simulink model "UiRlab6_model3"  (R2021a)
settings: Solver=VariableStepAuto  StartTime=0.0  StopTime=40e-3  RelTol=1e-3
undefined symbols (not defined in the file): K, Ka, Kf, Ki, Komega, Kria, Krsim, Kt, Ktr, Kzi, Ta, Tf_sim, Ti, Tii, Tisim, Tomega, Tt, Ttr, Tzi
settings Model: Creator=Luka  LastModifiedBy=Luka

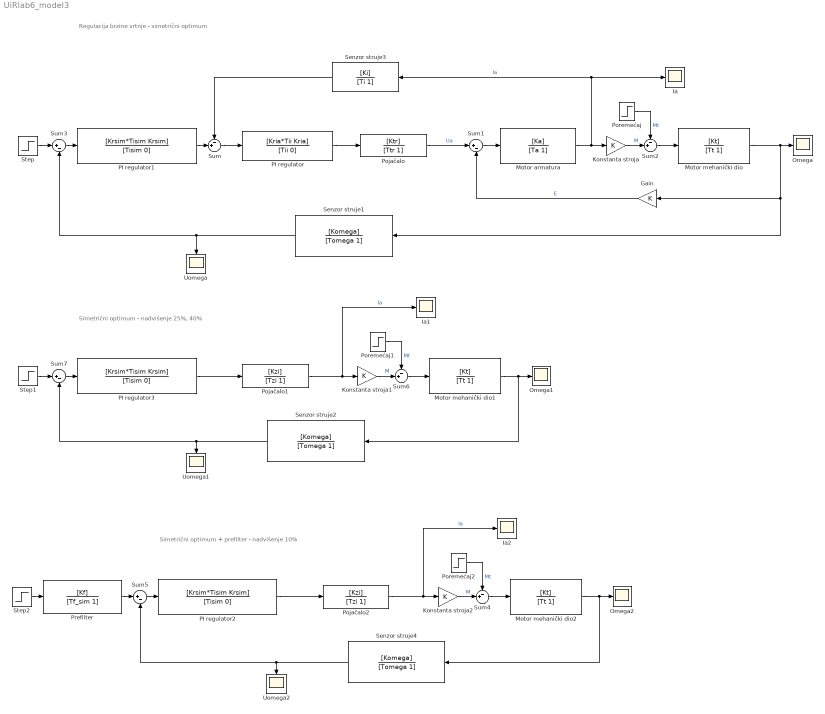
== system UiRlab6_model3 ==
  note: Simetrični optimum + prefilter - nadvišenje 10%
  note: Regulacija brzine vrtnje - simetrični optimum
  note: Simetrični optimum - nadvišenje 25%, 40%
  Gain : Gain  Gain=K
  Ia : Scope
  Ia1 : Scope
  Ia2 : Scope
  Konstanta stroja : Gain  Gain=K
  Konstanta stroja1 : Gain  Gain=K
  Konstanta stroja2 : Gain  Gain=K
  Motor armatura : TransferFcn  Numerator=[Ka]  Denominator=[Ta 1]
  Motor mehanički dio : TransferFcn  Numerator=[Kt]  Denominator=[Tt 1]
  Motor mehanički dio1 : TransferFcn  Numerator=[Kt]  Denominator=[Tt 1]
  Motor mehanički dio2 : TransferFcn  Numerator=[Kt]  Denominator=[Tt 1]
  Omega : Scope
  Omega1 : Scope
  Omega2 : Scope
  PI regulator : TransferFcn  Numerator=[Kria*Tii Kria]  Denominator=[Tii 0]
  PI regulator1 : TransferFcn  Numerator=[Krsim*Tisim Krsim]  Denominator=[Tisim 0]
  PI regulator2 : TransferFcn  Numerator=[Krsim*Tisim Krsim]  Denominator=[Tisim 0]
  PI regulator3 : TransferFcn  Numerator=[Krsim*Tisim Krsim]  Denominator=[Tisim 0]
  Pojačalo : TransferFcn  Numerator=[Ktr]  Denominator=[Ttr 1]
  Pojačalo1 : TransferFcn  Numerator=[Kzi]  Denominator=[Tzi 1]
  Pojačalo2 : TransferFcn  Numerator=[Kzi]  Denominator=[Tzi 1]
  Poremećaj : Step  Time=0  After=0  SampleTime=0
  Poremećaj1 : Step  Time=0  After=0  SampleTime=0
  Poremećaj2 : Step  Time=0  After=0  SampleTime=0
  Prefilter : TransferFcn  Numerator=[Kf]  Denominator=[Tf_sim 1]
  Senzor struje1 : TransferFcn  Numerator=[Komega]  Denominator=[Tomega 1]
  Senzor struje2 : TransferFcn  Numerator=[Komega]  Denominator=[Tomega 1]
  Senzor struje3 : TransferFcn  Numerator=[Ki]  Denominator=[Ti 1]
  Senzor struje4 : TransferFcn  Numerator=[Komega]  Denominator=[Tomega 1]
  Step : Step  Time=0  After=0.1  SampleTime=0
  Step1 : Step  Time=0  After=0.1  SampleTime=0
  Step2 : Step  Time=0  After=0.1  SampleTime=0
  Sum{,2,4,6} (4 alike) : Sum  Inputs=-+|
  Sum{1,3,5,7} (4 alike) : Sum  Inputs=|+-
  Uomega : Scope
  Uomega1 : Scope
  Uomega2 : Scope
  wires:
  Pojačalo1/1 -> Ia1/1, Konstanta stroja1/1  "Ia"
  Senzor struje1/1 -> Sum3/2, Uomega/1
  Step/1 -> Sum3/1
  PI regulator1/1 -> Sum/2
  Motor mehanički dio/1 -> Senzor struje1/1, Gain/1, Omega/1
  Konstanta stroja/1 -> Sum2/2  "M"
  Sum3/1 -> PI regulator1/1
  Senzor struje3/1 -> Sum/1
  PI regulator/1 -> Pojačalo/1
  Prefilter/1 -> Sum5/1
  Gain/1 -> Sum1/2  "E"
  Poremećaj/1 -> Sum2/1  "Mt"
  Sum6/1 -> Motor mehanički dio1/1
  Motor mehanički dio2/1 -> Omega2/1, Senzor struje4/1
  Pojačalo/1 -> Sum1/1  "Ua"
  Motor mehanički dio1/1 -> Omega1/1, Senzor struje2/1
  Sum7/1 -> PI regulator3/1
  Motor armatura/1 -> Senzor struje3/1, Ia/1, Konstanta stroja/1  "Ia"
  Sum/1 -> PI regulator/1
  Konstanta stroja1/1 -> Sum6/2  "M"
  Poremećaj2/1 -> Sum4/1  "Mt"
  Step1/1 -> Sum7/1
  Senzor struje2/1 -> Uomega1/1, Sum7/2
  Sum4/1 -> Motor mehanički dio2/1
  Pojačalo2/1 -> Ia2/1, Konstanta stroja2/1  "Ia"
  Senzor struje4/1 -> Uomega2/1, Sum5/2
  Step2/1 -> Prefilter/1
  Sum2/1 -> Motor mehanički dio/1
  Sum5/1 -> PI regulator2/1
  PI regulator2/1 -> Pojačalo2/1
  Sum1/1 -> Motor armatura/1
  PI regulator3/1 -> Pojačalo1/1
  Poremećaj1/1 -> Sum6/1  "Mt"
  Konstanta stroja2/1 -> Sum4/2  "M"
